simulink model "forward_converter"  (R2024b)
settings: Solver=VariableStepAuto  StartTime=0.0  StopTime=2  MaxStep=1e-4  RelTol=1e-4
libraries: spsMeanLib x5, spsVoltageMeasurementLib x5, spsCurrentMeasurementLib x4, spsDiodeLib x3, spsSeriesRLCBranchLib x3, spsDCVoltageSourceLib x1, spsGroundLib x1, spsLinearTransformerLib x1, spsMosfetLib x1, sps_lib x1
settings Model: Creator=m_pek  LastModifiedBy=m_pek

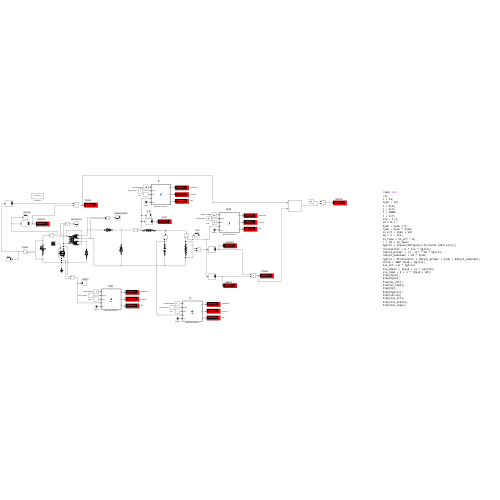
[thumbnail: Simulink's stored preview of the top-level diagram]
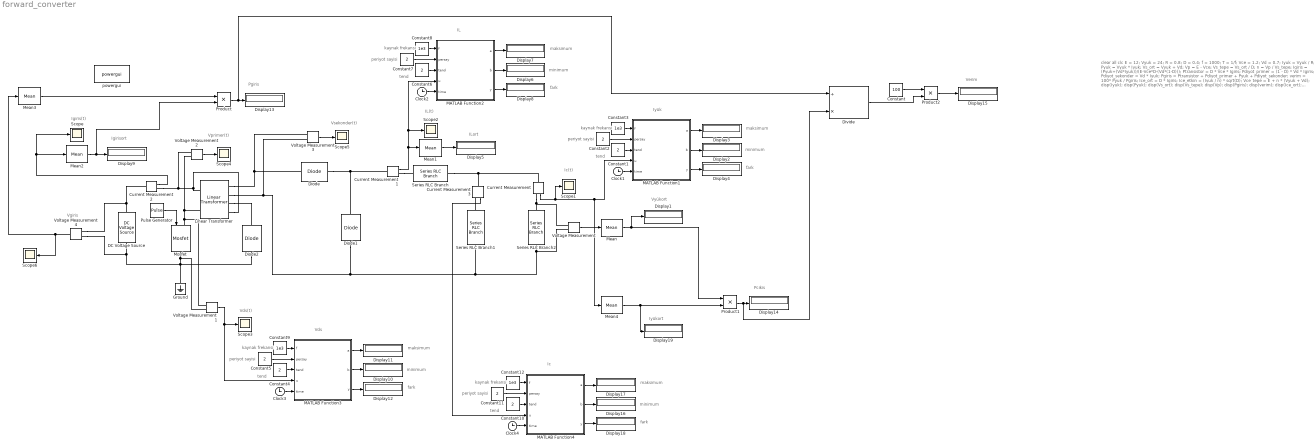
== system forward_converter ==
  note: clear all
      | clc
      | E = 12;
      | Vyuk = 24;
      | R = 0.8;
      | D = 0.4;
      | f = 1000;
      | T = 1/f;
      | Vce = 1.2;
      | Vd = 0.7;
      | Iyuk = Vyuk / R;
      | Pyuk = Vyuk * Iyuk;
      | Vs_ort = Vyuk + Vd;
      | Vp = E - Vce;
      | Vs_tepe = Vs_ort / D;
      | n = Vp / Vs_tepe;
      | Igiris = (Pyuk+(Vd*Iyuk))/(E-Vce*D-(Vd*(1-D)));
      | Ptransistor = D * Vce * Igiris;
      | Pdiyot_primer = (1 - D) * Vd * Igiris;
      | Pdiyot_sekonder = Vd * Iyuk;
      | Pgiris = Ptransistor + Pdiyot_primer + Pyuk + Pdiyot_sekonder;
      | verim = 100* Pyuk / Pgiris;
      | Ice_ort = D * Igiris;
      | Ice_etkin = (Iyuk / n) * sqrt(D);
      | Vce_tepe = E + n * (Vyuk + Vd);
      | disp(Iyuk);
      | disp(Pyuk);
      | disp(Vs_ort);
      | disp(Vs_tepe);
      | disp(Vp);
      | disp(Pgiris);
      | disp(verim);
      | disp(Ice_ort);
      | disp(Ice_etkin);
      | disp(Vce_tepe);
  note: Vyükort
  note: periyot sayisi
  note: maksimum
  note: fark
  note: minimum
  note: tend
  note: IL
  note: kaynak frekansi
  note: periyot sayisi
  note: maksimum
  note: fark
  note: minimum
  note: tend
  note: Iyük
  note: kaynak frekansi
  note: IL(t)
  note: Ic(t)
  note: Igiris(t)
  note: Igirisort
  note: ILort
  note: periyot sayisi
  note: maksimum
  note: fark
  note: minimum
  note: tend
  note: Vds
  note: kaynak frekansi
  note: Vds(t)
  note: Vprimer(t)
  note: Vsekonder(t)
  note: Pgiris
  note: Pcikis
  note: Vgiris
  note: kaynak frekansi
  note: periyot sayisi
  note: Ic
  note: tend
  note: fark
  note: maksimum
  note: minimum
  note: Verim
  note: Iyükort
  Clock{1..4} (4 alike) : Clock
      settings: Decimation=100
  Constant : Constant  Value=100
  Constant{1..2,4..7,10..11} (8 alike) : Constant  Value=2  SampleTime=0
  Constant{3,8..9,12} (4 alike) : Constant  Value=1e3  SampleTime=0
  Current Measurement{,1..3} (4 alike) : spsCurrentMeasurementLib/Current Measurement  PhasorSimulation=off  OutputType=Complex  PSBequivalent=0
  DC Voltage Source : spsDCVoltageSourceLib/DC Voltage Source  Amplitude=12  Measurements=None
  Diode : spsDiodeLib/Diode  Ron=0.001  Lon=0  Vf=0.7  IC=0  UseSnubber=0  Rs=500  Cs=250e-9  Measurements=off
  Diode1 : spsDiodeLib/Diode  Ron=0.001  Lon=0  Vf=0.7  IC=0  UseSnubber=0  Rs=500  Cs=250e-9  Measurements=off
  Diode2 : spsDiodeLib/Diode  Ron=0.001  Lon=0  Vf=0.7  IC=0  UseSnubber=0  Rs=500  Cs=250e-9  Measurements=off
  Display{1..19} (19 alike) : Display
  Divide : Product  Inputs=/*
  Ground : spsGroundLib/Ground  LConnTagsString=a
  Linear Transformer : spsLinearTransformerLib/Linear Transformer  UNITS=SI  NominalPower=[ 1000 1e3 ]  winding1=[100 0 0]  winding2=[500 0 0]  ThreeWindings=on  winding3=[100 0 0]  RmLm=[inf 1e-3]  Measurements=Magnetization current  DataType=on
  MATLAB Function1 : MATLAB Function  TreatAsAtomicUnit=on
  MATLAB Function2 : MATLAB Function  TreatAsAtomicUnit=on
  MATLAB Function3 : MATLAB Function  TreatAsAtomicUnit=on
  MATLAB Function4 : MATLAB Function  TreatAsAtomicUnit=on
  Mean{,1..4} (5 alike) : spsMeanLib/Mean  Freq=1e3  Vinit=0  Ts=0
  Mosfet : spsMosfetLib/Mosfet  Ron=0.1  Lon=0  Rd=1e-8  Vfd=1.2  IC=0  Rs=1e5  Cs=inf  Measurements=off
  Product : Product
  Product1 : Product
  Product2 : Product
  Pulse Generator : DiscretePulseGenerator  PulseType=Time based  Period=1/1e3  PulseWidth=40
  Scope{,1..6} (7 alike) : Scope
  Series RLC Branch : spsSeriesRLCBranchLib/Series RLC Branch  LConnTagsString=__new0  RConnTagsString=__new0  BranchType=L  Resistance=1  Inductance=4.8e-3  SetiL0=off  InitialCurrent=0  Capacitance=1e-6  Setx0=off  InitialVoltage=0  Measurements=None
  Series RLC Branch1 : spsSeriesRLCBranchLib/Series RLC Branch  LConnTagsString=__new0  RConnTagsString=__new0  BranchType=C  Resistance=1  Inductance=1e-3  SetiL0=off  InitialCurrent=0  Capacitance=100e-3  Setx0=off  InitialVoltage=0  Measurements=None
  Series RLC Branch2 : spsSeriesRLCBranchLib/Series RLC Branch  LConnTagsString=__new0  RConnTagsString=__new0  BranchType=R  Resistance=0.8  Inductance=1e-3  SetiL0=off  InitialCurrent=0  Capacitance=1e-6  Setx0=off  InitialVoltage=0  Measurements=None
  Voltage Measurement{,1..4} (5 alike) : spsVoltageMeasurementLib/Voltage Measurement  PhasorSimulation=off  OutputType=Complex  PSBequivalent=0
  powergui : sps_lib/powergui  Priority=1  SimulationMode=Continuous  SampleTime=50e-6  frequency=60  Iterations=50  frequencyindice=0  Pbase=100e6  ErrMax=1e-4  UnitsV=kV  UnitsW=MW  buscounter=0  FunctionMessages=off  echomessages=off  EnableUseOfTLC=off  CurrentSourceSwitches=off  DisableSnubberDevices=on  DisableRonSwitches=on  DisableVfSwitches=off  DisplayEquations=off  AutomaticDiscreteSolvers=off  SolverType=Tustin/Backward Euler (TBE)  Interpol=off  ExternalGateDelay=off  methode=off  Ts=100  x0status=blocks  SPID=on  SwTol=0  HookPort=off  NonlinearTolerance=1e-4  nMaxIteration=100  ContinueOnMaxIteration=off  RestoreLinks=warning  ResistiveCurrentMeasurement=off  Frange=[0:2:500]  Ylog=off  Xlog=on  ShowGrid=off  save=off  variable=ZData  structure=0  ZoomFFT=off  StartTime=0.0  cycles=1  DisplayStyle=1  fundamental=60  FreqAxis=off  MaxFrequency=1000  frequencyindicesteady=1  RmsSteady=1  display=off
  wires:
  Clock2/1 -> MATLAB Function2/5(time)
  Constant6/1 -> MATLAB Function2/3(tend)
  MATLAB Function2/3(y) -> Display8/1
  MATLAB Function2/2(b) -> Display6/1
  Voltage Measurement/1 -> Mean/1
  MATLAB Function2/1(a) -> Display7/1
  Constant8/1 -> MATLAB Function2/1(f)
  Constant7/1 -> MATLAB Function2/2(persay)
  Pulse Generator/1 -> Mosfet/1
  Mean/1 -> Product1/1, Display1/1
  Current Measurement1/1 -> Mean1/1, Scope2/1, MATLAB Function2/4(u)
  Current Measurement/1 -> Scope1/1, Mean4/1, MATLAB Function1/4(u)
  Constant2/1 -> MATLAB Function1/2(persay)
  Constant3/1 -> MATLAB Function1/1(f)
  MATLAB Function1/1(a) -> Display3/1
  MATLAB Function1/2(b) -> Display2/1
  MATLAB Function1/3(y) -> Display4/1
  Constant1/1 -> MATLAB Function1/3(tend)
  Clock1/1 -> MATLAB Function1/5(time)
  Mean1/1 -> Display5/1
  Mean2/1 -> Product/2, Display9/1
  Current Measurement2/1 -> Mean2/1, Scope/1
  Voltage Measurement1/1 -> MATLAB Function3/4(u), Scope3/1
  Constant5/1 -> MATLAB Function3/2(persay)
  Constant9/1 -> MATLAB Function3/1(f)
  MATLAB Function3/1(a) -> Display11/1
  MATLAB Function3/2(b) -> Display10/1
  MATLAB Function3/3(y) -> Display12/1
  Constant4/1 -> MATLAB Function3/3(tend)
  Clock3/1 -> MATLAB Function3/5(time)
  Voltage Measurement2/1 -> Scope4/1
  Voltage Measurement3/1 -> Scope5/1
  Product/1 -> Divide/1, Display13/1
  Product1/1 -> Divide/2, Display14/1
  Voltage Measurement4/1 -> Mean3/1, Scope6/1
  Mean3/1 -> Product/1
  Mean4/1 -> Display19/1, Product1/2
  Divide/1 -> Product2/2
  Constant/1 -> Product2/1
  Product2/1 -> Display15/1
  MATLAB Function4/2(b) -> Display16/1
  Constant12/1 -> MATLAB Function4/1(f)
  Constant11/1 -> MATLAB Function4/2(persay)
  Constant10/1 -> MATLAB Function4/3(tend)
  MATLAB Function4/1(a) -> Display17/1
  MATLAB Function4/3(y) -> Display18/1
  Clock4/1 -> MATLAB Function4/5(time)
  Current Measurement3/1 -> MATLAB Function4/4(u)
  connections:
  DC Voltage Source/RConn1 -- Voltage Measurement4/LConn1 -- Current Measurement2/LConn1
  Mosfet/LConn1 -- Linear Transformer/LConn2 -- Voltage Measurement2/LConn2 -- Voltage Measurement1/LConn1
  Linear Transformer/RConn1 -- Diode/LConn1 -- Voltage Measurement3/LConn1
  Diode/RConn1 -- Current Measurement1/LConn1 -- Diode1/RConn1
  Current Measurement3/RConn1 -- Series RLC Branch1/LConn1
  Diode1/LConn1 -- Linear Transformer/RConn2 -- Voltage Measurement3/LConn2 -- Series RLC Branch1/RConn1 -- Voltage Measurement/LConn2 -- Series RLC Branch2/RConn1
  Mosfet/RConn1 -- Ground/LConn1 -- Voltage Measurement4/LConn2 -- DC Voltage Source/LConn1 -- Diode2/LConn1 -- Voltage Measurement1/LConn2
  Voltage Measurement/LConn1 -- Current Measurement/RConn1 -- Series RLC Branch2/LConn1
  Current Measurement1/RConn1 -- Series RLC Branch/LConn1
  Current Measurement2/RConn1 -- Voltage Measurement2/LConn1 -- Linear Transformer/RConn4 -- Linear Transformer/LConn1
  Linear Transformer/RConn3 -- Diode2/RConn1
  Series RLC Branch/RConn1 -- Current Measurement/LConn1 -- Current Measurement3/LConn1

== matlab function forward_converter/MATLAB Function1 ==
  settings: updateMethod=DISCRETE  sampleTime=50e-8
  data: a output; b output; f input; persay input; tend input; u input; y output; time input
function [a,b,y] = fcn(f,persay,tend,u,time)
% persistent değişken; değişken değerini kalıcı olarak tutar ve direk atama
% yapılmadıkça değişmez. Normal değişkenler fonksiyonun her yenilenme 
% durumunda sıfırlanırken, persistent değişkeni, kalıcı olması sebebiyle,
% bir önceki değeri tutabilme yeteneğine sahiptir. 
% Bu da bize bir önceki değer ile güncel değerinizi karşılaştırma olanağı
% sunar.
a=1/0;b=0;
persistent enbuyuk;
persistent enkucuk;
persistent fark;
% Eğer persistent değişkenini en başta persistent enbuyuk = 0; olarak 
% tanımlarsak, sürekli 0 olarak kalacaktır. Aynı zamanda eğer bir ilk değer 
% vermezseniz "null" değerini taşıyacağından, if yapılarında hata
% verecektir. Bu hatadan kaçınmak için, isempty komutu ile persistent
% değişkenlerinin "null" olup olmadığını kontrol edilir ve ilk değer ataması
% yapılır. Bu değişkenler sadece  fonksiyon ilk kez çalıştığında
% null olacağı için(daha sonra sürekli gelen değeri tuttuğu yukarıda söylenmişti)
% başlangıçta, bir kereye mahsus olarak,  aşağıdaki if yapısı doğrulanacak 
% ve değişkenlere ilk değerler atanacaktır.
%
if (isempty(enkucuk) || isempty(enbuyuk))  
enkucuk = 1/0;   
enbuyuk = 0;
end
if (time>tend-(persay+1)*1/f) && (time<=tend) % Periyot ~= 0.01 // Son iki periyodu hesaplar.
    if u >= enbuyuk
        enbuyuk = u;
     end
    if u < enkucuk   
        enkucuk = u;
    end
end
fark = enbuyuk - enkucuk;
a=enbuyuk;
b=enkucuk;
y=fark;
end

== matlab function forward_converter/MATLAB Function3 ==
  settings: updateMethod=DISCRETE  sampleTime=50e-8
  data: a output; b output; f input; persay input; tend input; u input; y output; time input
function [a,b,y] = fcn(f,persay,tend,u,time)
% persistent değişken; değişken değerini kalıcı olarak tutar ve direk atama
% yapılmadıkça değişmez. Normal değişkenler fonksiyonun her yenilenme 
% durumunda sıfırlanırken, persistent değişkeni, kalıcı olması sebebiyle,
% bir önceki değeri tutabilme yeteneğine sahiptir. 
% Bu da bize bir önceki değer ile güncel değerinizi karşılaştırma olanağı
% sunar.
a=1/0;b=0;
persistent enbuyuk;
persistent enkucuk;
persistent fark;
% Eğer persistent değişkenini en başta persistent enbuyuk = 0; olarak 
% tanımlarsak, sürekli 0 olarak kalacaktır. Aynı zamanda eğer bir ilk değer 
% vermezseniz "null" değerini taşıyacağından, if yapılarında hata
% verecektir. Bu hatadan kaçınmak için, isempty komutu ile persistent
% değişkenlerinin "null" olup olmadığını kontrol edilir ve ilk değer ataması
% yapılır. Bu değişkenler sadece  fonksiyon ilk kez çalıştığında
% null olacağı için(daha sonra sürekli gelen değeri tuttuğu yukarıda söylenmişti)
% başlangıçta, bir kereye mahsus olarak,  aşağıdaki if yapısı doğrulanacak 
% ve değişkenlere ilk değerler atanacaktır.
%
if (isempty(enkucuk) || isempty(enbuyuk))  
enkucuk = 1/0;   
enbuyuk = 0;
end
if (time>tend-(persay+1)*1/f) && (time<=tend) % Periyot ~= 0.01 // Son iki periyodu hesaplar.
    if u >= enbuyuk
        enbuyuk = u;
     end
    if u < enkucuk   
        enkucuk = u;
    end
end
fark = enbuyuk - enkucuk;
a=enbuyuk;
b=enkucuk;
y=fark;
end

== matlab function forward_converter/MATLAB Function2 ==
  settings: updateMethod=DISCRETE  sampleTime=50e-8
  data: a output; b output; f input; persay input; tend input; u input; y output; time input
function [a,b,y] = fcn(f,persay,tend,u,time)
% persistent değişken; değişken değerini kalıcı olarak tutar ve direk atama
% yapılmadıkça değişmez. Normal değişkenler fonksiyonun her yenilenme 
% durumunda sıfırlanırken, persistent değişkeni, kalıcı olması sebebiyle,
% bir önceki değeri tutabilme yeteneğine sahiptir. 
% Bu da bize bir önceki değer ile güncel değerinizi karşılaştırma olanağı
% sunar.
a=1/0;b=0;
persistent enbuyuk;
persistent enkucuk;
persistent fark;
% Eğer persistent değişkenini en başta persistent enbuyuk = 0; olarak 
% tanımlarsak, sürekli 0 olarak kalacaktır. Aynı zamanda eğer bir ilk değer 
% vermezseniz "null" değerini taşıyacağından, if yapılarında hata
% verecektir. Bu hatadan kaçınmak için, isempty komutu ile persistent
% değişkenlerinin "null" olup olmadığını kontrol edilir ve ilk değer ataması
% yapılır. Bu değişkenler sadece  fonksiyon ilk kez çalıştığında
% null olacağı için(daha sonra sürekli gelen değeri tuttuğu yukarıda söylenmişti)
% başlangıçta, bir kereye mahsus olarak,  aşağıdaki if yapısı doğrulanacak 
% ve değişkenlere ilk değerler atanacaktır.
%
if (isempty(enkucuk) || isempty(enbuyuk))  
enkucuk = 1/0;   
enbuyuk = 0;
end
if (time>tend-(persay+1)*1/f) && (time<=tend) % Periyot ~= 0.01 // Son iki periyodu hesaplar.
    if u >= enbuyuk
        enbuyuk = u;
     end
    if u < enkucuk   
        enkucuk = u;
    end
end
fark = enbuyuk - enkucuk;
a=enbuyuk;
b=enkucuk;
y=fark;
end

== matlab function forward_converter/MATLAB Function4 ==
  settings: updateMethod=DISCRETE  sampleTime=50e-8
  data: a output; b output; f input; persay input; tend input; u input; y output; time input
function [a,b,y] = fcn(f,persay,tend,u,time)
% persistent değişken; değişken değerini kalıcı olarak tutar ve direk atama
% yapılmadıkça değişmez. Normal değişkenler fonksiyonun her yenilenme 
% durumunda sıfırlanırken, persistent değişkeni, kalıcı olması sebebiyle,
% bir önceki değeri tutabilme yeteneğine sahiptir. 
% Bu da bize bir önceki değer ile güncel değerinizi karşılaştırma olanağı
% sunar.
a=1/0;b=0;
persistent enbuyuk;
persistent enkucuk;
persistent fark;
% Eğer persistent değişkenini en başta persistent enbuyuk = 0; olarak 
% tanımlarsak, sürekli 0 olarak kalacaktır. Aynı zamanda eğer bir ilk değer 
% vermezseniz "null" değerini taşıyacağından, if yapılarında hata
% verecektir. Bu hatadan kaçınmak için, isempty komutu ile persistent
% değişkenlerinin "null" olup olmadığını kontrol edilir ve ilk değer ataması
% yapılır. Bu değişkenler sadece  fonksiyon ilk kez çalıştığında
% null olacağı için(daha sonra sürekli gelen değeri tuttuğu yukarıda söylenmişti)
% başlangıçta, bir kereye mahsus olarak,  aşağıdaki if yapısı doğrulanacak 
% ve değişkenlere ilk değerler atanacaktır.
%
if (isempty(enkucuk) || isempty(enbuyuk))  
enkucuk = 1/0;   
enbuyuk = 0;
end
if (time>tend-(persay+1)*1/f) && (time<=tend) % Periyot ~= 0.01 // Son iki periyodu hesaplar.
    if u >= enbuyuk
        enbuyuk = u;
     end
    if u < enkucuk   
        enkucuk = u;
    end
end
fark = enbuyuk - enkucuk;
a=enbuyuk;
b=enkucuk;
y=fark;
end
